simulink model "project_to_axes"  (R2018a)
settings: Solver=VariableStepAuto  StartTime=0.0  StopTime=10.0  RelTol=1e-3
settings Model: Creator=Rafael  LastModifiedBy=Rafael
settings DataIOCC: SaveOutput=off  SaveTime=off

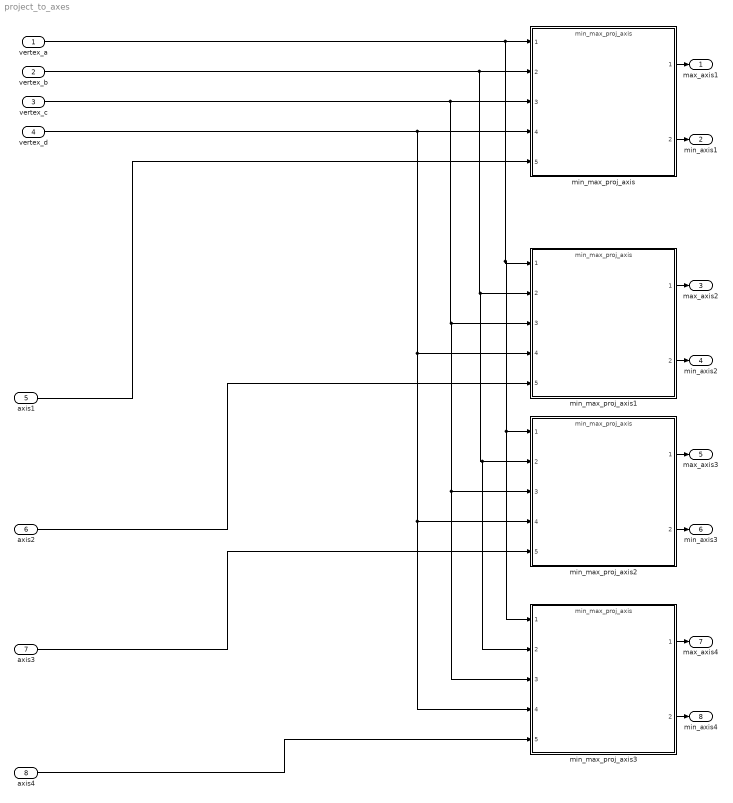
== system project_to_axes ==
  vertex_a : Inport  OutDataTypeStr=double  PortDimensions=2  SampleTime=0
  vertex_b : Inport  Port=2  OutDataTypeStr=double  PortDimensions=2  SampleTime=0
  vertex_c : Inport  Port=3  OutDataTypeStr=double  PortDimensions=2  SampleTime=0
  vertex_d : Inport  Port=4  OutDataTypeStr=double  PortDimensions=2  SampleTime=0
  axis1 : Inport  Port=5  OutDataTypeStr=double  PortDimensions=2  SampleTime=0
  axis2 : Inport  Port=6  OutDataTypeStr=double  PortDimensions=2  SampleTime=0
  axis3 : Inport  Port=7  OutDataTypeStr=double  PortDimensions=2  SampleTime=0
  axis4 : Inport  Port=8  OutDataTypeStr=double  PortDimensions=2  SampleTime=0
  min_max_proj_axis{,1..3} (4 alike) : ModelReference  ModelNameDialog=min_max_proj_axis  SimulationMode=Normal  ModelReferenceVersion=1.18
  max_axis1 : Outport  OutDataTypeStr=double  PortDimensions=1  SampleTime=0
  min_axis1 : Outport  Port=2  OutDataTypeStr=double  PortDimensions=1  SampleTime=0
  max_axis2 : Outport  Port=3  OutDataTypeStr=double  PortDimensions=1  SampleTime=0
  min_axis2 : Outport  Port=4  OutDataTypeStr=double  PortDimensions=1  SampleTime=0
  max_axis3 : Outport  Port=5  OutDataTypeStr=double  PortDimensions=1  SampleTime=0
  min_axis3 : Outport  Port=6  OutDataTypeStr=double  PortDimensions=1  SampleTime=0
  max_axis4 : Outport  Port=7  OutDataTypeStr=double  PortDimensions=1  SampleTime=0
  min_axis4 : Outport  Port=8  OutDataTypeStr=double  PortDimensions=1  SampleTime=0
  wires:
  vertex_c/1 -> min_max_proj_axis/3, min_max_proj_axis1/3, min_max_proj_axis2/3, min_max_proj_axis3/3
  min_max_proj_axis/1 -> max_axis1/1
  vertex_a/1 -> min_max_proj_axis/1, min_max_proj_axis1/1, min_max_proj_axis2/1, min_max_proj_axis3/1
  vertex_d/1 -> min_max_proj_axis/4, min_max_proj_axis1/4, min_max_proj_axis2/4, min_max_proj_axis3/4
  min_max_proj_axis/2 -> min_axis1/1
  min_max_proj_axis3/2 -> min_axis4/1
  min_max_proj_axis2/2 -> min_axis3/1
  axis3/1 -> min_max_proj_axis2/5
  vertex_b/1 -> min_max_proj_axis/2, min_max_proj_axis1/2, min_max_proj_axis2/2, min_max_proj_axis3/2
  min_max_proj_axis1/1 -> max_axis2/1
  min_max_proj_axis3/1 -> max_axis4/1
  axis2/1 -> min_max_proj_axis1/5
  axis1/1 -> min_max_proj_axis/5
  axis4/1 -> min_max_proj_axis3/5
  min_max_proj_axis1/2 -> min_axis2/1
  min_max_proj_axis2/1 -> max_axis3/1
